simulink model "main_SEPETC"  (R2021a)
settings: Solver=VariableStepAuto  StartTime=0.0  StopTime=10  RelTol=1e-3
InitFcn:
  | run('Parameter.m')
values from neighbouring files (symbols this model uses):
  cp = 1    [Parameter.m]
  cv = 5    [Parameter.m]
  cw = 5    [Parameter.m]
  fref = 60    [Parameter.m]
  Lc1 = 0.35e-3    (= 0.00035)    [Parameter.m]
  Lc2 = 0.35e-3    (= 0.00035)    [Parameter.m]
  Lc3 = 0.35e-3    (= 0.00035)    [Parameter.m]
  Lc4 = 0.35e-3    (= 0.00035)    [Parameter.m]
  Lt12 = 318e-6    (= 0.000318)    [Parameter.m]
  Lt23 = 1847e-6    (= 0.001847)    [Parameter.m]
  Lt34 = 318e-6    (= 0.000318)    [Parameter.m]
  Mp1 = 9.4e-5    (= 9.4e-05)    [Parameter.m]
  Mp2 = 9.4e-5    (= 9.4e-05)    [Parameter.m]
  Mp3 = 12.5e-5    (= 0.000125)    [Parameter.m]
  Mp4 = 12.5e-5    (= 0.000125)    [Parameter.m]
  Nq1 = 1.3e-3    (= 0.0013)    [Parameter.m]
  Nq2 = 1.3e-3    (= 0.0013)    [Parameter.m]
  Nq3 = 1.5e-3    (= 0.0015)    [Parameter.m]
  Nq4 = 1.5e-3    (= 0.0015)    [Parameter.m]
  Rc1 = 0.03    [Parameter.m]
  Rc2 = 0.03    [Parameter.m]
  Rc3 = 0.03    [Parameter.m]
  Rc4 = 0.03    [Parameter.m]
  Rt12 = 0.23    [Parameter.m]
  Rt23 = 0.35    [Parameter.m]
  Rt34 = 0.23    [Parameter.m]
  t2 = 1    [Parameter.m]    (also in wvp_SEPETC.m)
  t3 = 10    [Parameter.m]
  t4 = 20    [Parameter.m]    (also in wvp_SEPETC.m = 21)
  t5 = 35    [Parameter.m]    (also in wvp_SEPETC.m = 33)
  t6 = 40    [Parameter.m]    (also in wvp_SEPETC.m = 35)
  Uo = 220*sqrt(2)    [Parameter.m]
  vref = 380    [Parameter.m]
  wc = 31.4    [Parameter.m]
  wref = 2*pi*fref    (= 376.991118431)    [Parameter.m]
undefined symbols (not defined in the file or in its folder): gcbh, sps_rtmsupport
libraries: spsControlledVoltageSourceLib x12, spsAlphaBetaZerotodq0Lib x12, eeGeneralControl x8, spsThreePhaseSeriesRLCBranchLib x7, spsGroundLib x4, spsThreePhaseVIMeasurementLib x4, spsThreePhaseBreakerLib x4, spsPLL3phLib x4, spsThreePhaseSeriesRLCLoadLib x3, spspowerguiLib x1
(part 2 of 3)

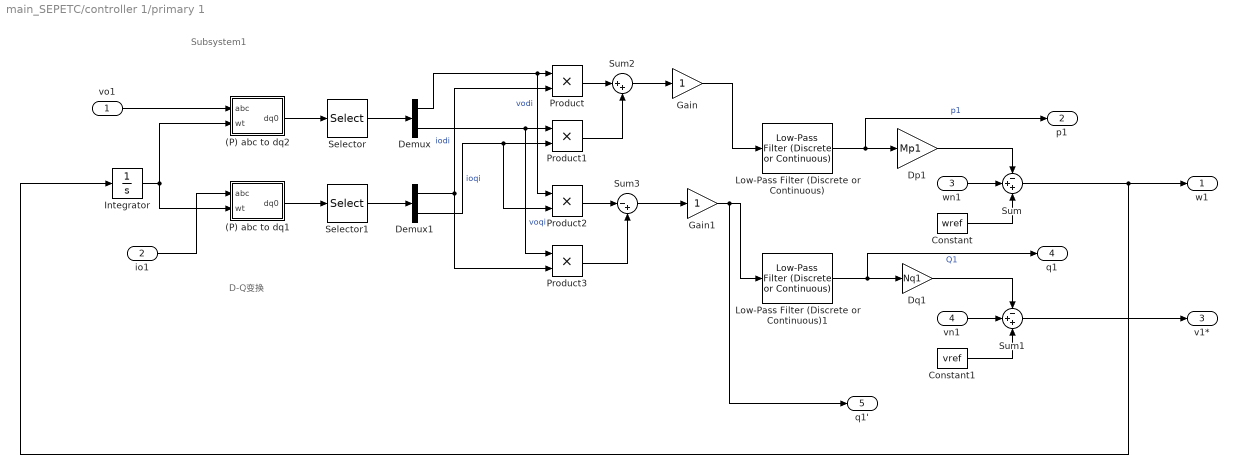
== system main_SEPETC/controller 1/primary 1 ==
  note: Subsystem1
  note: D-Q变换
  vo1 : Inport
  io1 : Inport  Port=2
  wn1 : Inport  Port=3
  vn1 : Inport  Port=4
  (P) abc to dq1 : Subsystem  AncestorBlock=powerlib_meascontrol/Transformations/abc to dq0  DialogController=POWERSYS.PowerSysDialog  LoadFcn=sps_rtmsupport('LoadFcn', gcbh);  StartFcn=sps_rtmsupport('StartFcn', gcbh);  StopFcn=sps_rtmsupport('StopFcn', gcbh);  mask(abc to dq0 Transformation){Alignment=90 degrees behind phase A axis}
      mask prompts: Alignment "Rotating frame alignment at wt=0:"
      mask help:
      | Perform a Park transformation from a three-phase (abc) signal to a dq0 rotating reference frame. Angular position of the rotating frame is given by input wt (rad).
      |
      | When the rotating frame alignment at wt=0 is 90 degrees behind phase A axis, a positive-sequence signal with Mag=1 & Phase=0 degrees yields the following dq values: d=1, q=0.
      mask init:
      | str=cat(2,gcb,'/Alpha-Beta-Zero to dq0');
      | if Alignment==1
      |     set_param(str,'Alignment','Aligned with phase A axis');
      | else
      |     set_param(str,'Alignment','90 degrees behind phase A axis');
      | end
      settings: CopyFcn=sps_rtmsupport('CopyFcn', gcbh);  DeleteFcn=sps_rtmsupport('DeleteFcn', gcbh);  UndoDeleteFcn=sps_rtmsupport('UndoDeleteFcn', gcbh);  ModelCloseFcn=sps_rtmsupport('ModelCloseFcn', gcbh);  PreSaveFcn=sps_rtmsupport('PreSaveFcn', gcbh);  PostSaveFcn=sps_rtmsupport('PostSaveFcn', gcbh);  NameChangeFcn=sps_rtmsupport('NameChangeFcn', gcbh);  PreCopyFcn=sps_rtmsupport('PreCopyFcn', gcbh);  OpenFcn=sps_rtmsupport('OpenFcn', gcbh, [1]);  CloseFcn=sps_rtmsupport('CloseFcn', gcbh);  PreDeleteFcn=sps_rtmsupport('PreDeleteFcn', gcbh);
      mask Help: helpview(psbhelp);
      mask TypeOptions Alignment: Aligned with phase A axis | 90 degrees behind phase A axis
      mask Display:
      | plot([0 1], [0,1])
      | port_label('input', 1, 'abc')
      | port_label('input', 2, 'wt')
      | port_label('output', 1, 'dq0')
  (P) abc to dq2 : Subsystem  AncestorBlock=powerlib_meascontrol/Transformations/abc to dq0  DialogController=POWERSYS.PowerSysDialog  LoadFcn=sps_rtmsupport('LoadFcn', gcbh);  StartFcn=sps_rtmsupport('StartFcn', gcbh);  StopFcn=sps_rtmsupport('StopFcn', gcbh);  mask(abc to dq0 Transformation){Alignment=90 degrees behind phase A axis}
      mask prompts: Alignment "Rotating frame alignment at wt=0:"
      mask help:
      | Perform a Park transformation from a three-phase (abc) signal to a dq0 rotating reference frame. Angular position of the rotating frame is given by input wt (rad).
      |
      | When the rotating frame alignment at wt=0 is 90 degrees behind phase A axis, a positive-sequence signal with Mag=1 & Phase=0 degrees yields the following dq values: d=1, q=0.
      mask init:
      | str=cat(2,gcb,'/Alpha-Beta-Zero to dq0');
      | if Alignment==1
      |     set_param(str,'Alignment','Aligned with phase A axis');
      | else
      |     set_param(str,'Alignment','90 degrees behind phase A axis');
      | end
      settings: CopyFcn=sps_rtmsupport('CopyFcn', gcbh);  DeleteFcn=sps_rtmsupport('DeleteFcn', gcbh);  UndoDeleteFcn=sps_rtmsupport('UndoDeleteFcn', gcbh);  ModelCloseFcn=sps_rtmsupport('ModelCloseFcn', gcbh);  PreSaveFcn=sps_rtmsupport('PreSaveFcn', gcbh);  PostSaveFcn=sps_rtmsupport('PostSaveFcn', gcbh);  NameChangeFcn=sps_rtmsupport('NameChangeFcn', gcbh);  PreCopyFcn=sps_rtmsupport('PreCopyFcn', gcbh);  OpenFcn=sps_rtmsupport('OpenFcn', gcbh, [1]);  CloseFcn=sps_rtmsupport('CloseFcn', gcbh);  PreDeleteFcn=sps_rtmsupport('PreDeleteFcn', gcbh);
      mask Help: helpview(psbhelp);
      mask TypeOptions Alignment: Aligned with phase A axis | 90 degrees behind phase A axis
      mask Display:
      | plot([0 1], [0,1])
      | port_label('input', 1, 'abc')
      | port_label('input', 2, 'wt')
      | port_label('output', 1, 'dq0')
  Constant : Constant  Value=wref
  Constant1 : Constant  Value=vref
  Demux : Demux  Outputs=2
  Demux1 : Demux  Outputs=2
  Dp1 : Gain  Gain=Mp1
  Dq1 : Gain  Gain=Nq1
  Gain : Gain
  Gain1 : Gain
  Integrator : Integrator
  Low-Pass Filter (Discrete or Continuous) : eeGeneralControl/Low-Pass Filter (Discrete or Continuous)  K=1  T=1/wc  B=inf  A=-inf  init_option=Inherited from block input  x0=0  Ts=-1
  Low-Pass Filter (Discrete or Continuous)1 : eeGeneralControl/Low-Pass Filter (Discrete or Continuous)  K=1  T=1/wc  B=inf  A=-inf  init_option=Inherited from block input  x0=0  Ts=-1
  Product{,1..3} (4 alike) : Product
  Selector : Selector  InputPortWidth=3  IndexOptions=Index vector (dialog)  Indices=[1 2]  OutputSizes=1
  Selector1 : Selector  InputPortWidth=3  IndexOptions=Index vector (dialog)  Indices=[1 2]  OutputSizes=1
  Sum : Sum  Inputs=-++
  Sum1 : Sum  Inputs=-++
  Sum2 : Sum  Inputs=|++
  Sum3 : Sum  Inputs=|-+
  w1 : Outport
  p1 : Outport  Port=2
  v1* : Outport  Port=3
  q1 : Outport  Port=4
  q1' : Outport  Port=5
  wires:
  Low-Pass Filter (Discrete or Continuous)/1 -> Dp1/1, p1/1  "p1"
  Dp1/1 -> Sum/1
  wn1/1 -> Sum/2
  Sum/1 -> Integrator/1, w1/1
  Dq1/1 -> Sum1/1
  Low-Pass Filter (Discrete or Continuous)1/1 -> Dq1/1, q1/1  "Q1"
  Sum1/1 -> v1*/1
  vn1/1 -> Sum1/2
  Constant1/1 -> Sum1/3
  Constant/1 -> Sum/3
  Gain1/1 -> q1'/1, Low-Pass Filter (Discrete or Continuous)1/1
  Gain/1 -> Low-Pass Filter (Discrete or Continuous)/1
  Sum3/1 -> Gain1/1
  Sum2/1 -> Gain/1
  vo1/1 -> (P) abc to dq2/1(abc)
  io1/1 -> (P) abc to dq1/1(abc)
  Product/1 -> Sum2/1
  Product1/1 -> Sum2/2
  Demux1/2 -> Product1/2, Product2/2  "ioqi"
  Product2/1 -> Sum3/1
  Product3/1 -> Sum3/2
  (P) abc to dq1/1(dq0) -> Selector1/1
  Demux1/1 -> Product3/2, Product/2  "iodi"
  (P) abc to dq2/1(dq0) -> Selector/1
  Demux/1 -> Product2/1, Product/1  "vodi"
  Integrator/1 -> (P) abc to dq1/2(wt), (P) abc to dq2/2(wt)
  Selector1/1 -> Demux1/1
  Demux/2 -> Product1/1, Product3/1  "voqi"
  Selector/1 -> Demux/1

== system main_SEPETC/controller 1/v_secondary 1 ==
  q1' : Inport
  Constant : Constant  Value=wc
  Gain1 : Gain  Gain=wc
  Gain11 : Gain  Gain=Nq1
  Gain5 : Gain  Gain=cv
  Integrator : Integrator  ExternalReset=rising
  Product : Product
  Step : Step  Time=t2  SampleTime=0
  Sum : Sum  Inputs=|+-
  Sum5 : Sum  Inputs=|++
  vn1 : Outport
  wires:
  [zv1] -> Gain5/1
  q1'/1 -> Product/1
  Constant/1 -> Product/2
  Product/1 -> Sum/1
  Gain1/1 -> Sum/2
  [q1] -> Gain1/1
  Sum/1 -> Gain11/1
  Gain5/1 -> Sum5/1
  Gain11/1 -> Sum5/2
  Sum5/1 -> Integrator/1
  Step/1 -> Integrator/2
  Integrator/1 -> vn1/1

== system main_SEPETC/controller 1/w_secondary 1 ==
  Gain : Gain  Gain=cw
  Gain15 : Gain  Gain=cp
  Integrator : Integrator  ExternalReset=rising
  Step : Step  Time=t2  SampleTime=0
  Sum6 : Sum  Inputs=++|
  wn1 : Outport
  wires:
  Sum6/1 -> Integrator/1
  Gain15/1 -> Sum6/2
  Integrator/1 -> wn1/1
  [zw1] -> Gain/1
  Gain/1 -> Sum6/1
  [zp1] -> Gain15/1
  Step/1 -> Integrator/2

== system main_SEPETC/controller 2/(P) abc to dq2 ==
  abc : Inport  PortDimensions=3
  wt : Inport  Port=2  PortDimensions=1
  Alpha-Beta-Zero to dq0 : spsAlphaBetaZerotodq0Lib/Alpha-Beta-Zero to dq0  Alignment=90 degrees behind phase A axis
      settings: SourceProductBaseCode=PS
  abc to Alpha-Beta-Zero : Subsystem  AncestorBlock=powerlib_meascontrol/Transformations/abc to Alpha-Beta-Zero  DialogController=POWERSYS.PowerSysDialog  LoadFcn=sps_rtmsupport('LoadFcn', gcbh);  StartFcn=sps_rtmsupport('StartFcn', gcbh);  StopFcn=sps_rtmsupport('StopFcn', gcbh);  mask(abc to Alpha-Beta-Zero Transformation){}
      mask help: Perform a Clarke transformation from a three-phase (abc) signal to a alpha-beta-zero stationary reference frame.
      settings: CopyFcn=sps_rtmsupport('CopyFcn', gcbh);  DeleteFcn=sps_rtmsupport('DeleteFcn', gcbh);  UndoDeleteFcn=sps_rtmsupport('UndoDeleteFcn', gcbh);  ModelCloseFcn=sps_rtmsupport('ModelCloseFcn', gcbh);  PreSaveFcn=sps_rtmsupport('PreSaveFcn', gcbh);  PostSaveFcn=sps_rtmsupport('PostSaveFcn', gcbh);  NameChangeFcn=sps_rtmsupport('NameChangeFcn', gcbh);  PreCopyFcn=sps_rtmsupport('PreCopyFcn', gcbh);  OpenFcn=sps_rtmsupport('OpenFcn', gcbh, []);  CloseFcn=sps_rtmsupport('CloseFcn', gcbh);  PreDeleteFcn=sps_rtmsupport('PreDeleteFcn', gcbh);
      mask Help: helpview(psbhelp);
      mask Display:
      | plot([0 1], [0,1])
      | text(0.15,0.7,'abc')
      | text(0.55, 0.3,'\alpha\beta0','texmode','on')
  dq0 : Outport  VectorParamsAs1DForOutWhenUnconnected=off
  wires:
  wt/1 -> Alpha-Beta-Zero to dq0/2
  abc/1 -> abc to Alpha-Beta-Zero/1(abc)
  Alpha-Beta-Zero to dq0/1 -> dq0/1
  abc to Alpha-Beta-Zero/1(al_be_0) -> Alpha-Beta-Zero to dq0/1

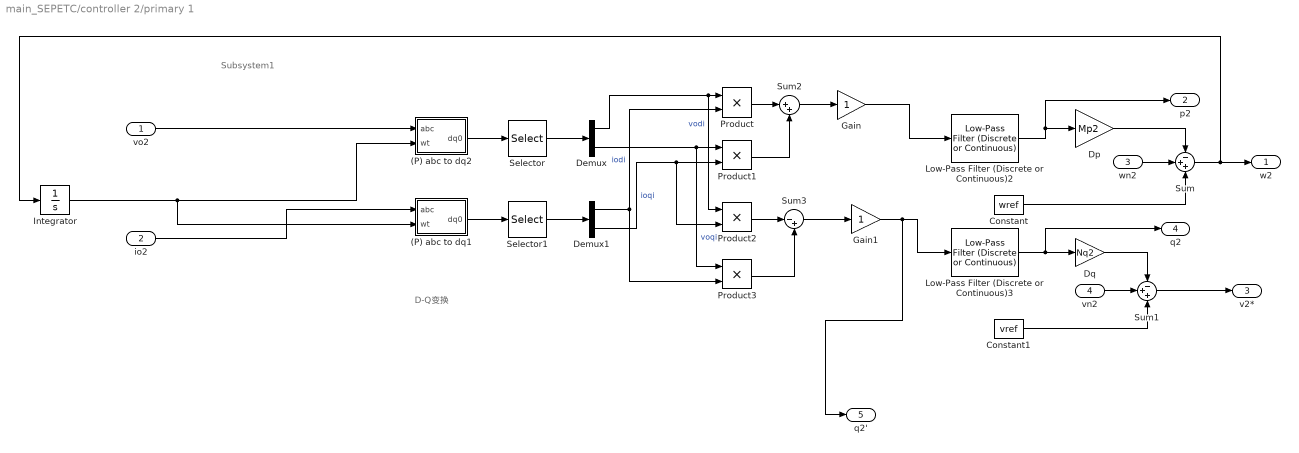
== system main_SEPETC/controller 2/primary 1 ==
  note: Subsystem1
  note: D-Q变换
  vo2 : Inport
  io2 : Inport  Port=2
  wn2 : Inport  Port=3
  vn2 : Inport  Port=4
  (P) abc to dq1 : Subsystem  AncestorBlock=powerlib_meascontrol/Transformations/abc to dq0  DialogController=POWERSYS.PowerSysDialog  LoadFcn=sps_rtmsupport('LoadFcn', gcbh);  StartFcn=sps_rtmsupport('StartFcn', gcbh);  StopFcn=sps_rtmsupport('StopFcn', gcbh);  mask(abc to dq0 Transformation){Alignment=90 degrees behind phase A axis}
      mask prompts: Alignment "Rotating frame alignment at wt=0:"
      mask help:
      | Perform a Park transformation from a three-phase (abc) signal to a dq0 rotating reference frame. Angular position of the rotating frame is given by input wt (rad).
      |
      | When the rotating frame alignment at wt=0 is 90 degrees behind phase A axis, a positive-sequence signal with Mag=1 & Phase=0 degrees yields the following dq values: d=1, q=0.
      mask init:
      | str=cat(2,gcb,'/Alpha-Beta-Zero to dq0');
      | if Alignment==1
      |     set_param(str,'Alignment','Aligned with phase A axis');
      | else
      |     set_param(str,'Alignment','90 degrees behind phase A axis');
      | end
      settings: CopyFcn=sps_rtmsupport('CopyFcn', gcbh);  DeleteFcn=sps_rtmsupport('DeleteFcn', gcbh);  UndoDeleteFcn=sps_rtmsupport('UndoDeleteFcn', gcbh);  ModelCloseFcn=sps_rtmsupport('ModelCloseFcn', gcbh);  PreSaveFcn=sps_rtmsupport('PreSaveFcn', gcbh);  PostSaveFcn=sps_rtmsupport('PostSaveFcn', gcbh);  NameChangeFcn=sps_rtmsupport('NameChangeFcn', gcbh);  PreCopyFcn=sps_rtmsupport('PreCopyFcn', gcbh);  OpenFcn=sps_rtmsupport('OpenFcn', gcbh, [1]);  CloseFcn=sps_rtmsupport('CloseFcn', gcbh);  PreDeleteFcn=sps_rtmsupport('PreDeleteFcn', gcbh);
      mask Help: helpview(psbhelp);
      mask TypeOptions Alignment: Aligned with phase A axis | 90 degrees behind phase A axis
      mask Display:
      | plot([0 1], [0,1])
      | port_label('input', 1, 'abc')
      | port_label('input', 2, 'wt')
      | port_label('output', 1, 'dq0')
  (P) abc to dq2 : Subsystem  AncestorBlock=powerlib_meascontrol/Transformations/abc to dq0  DialogController=POWERSYS.PowerSysDialog  LoadFcn=sps_rtmsupport('LoadFcn', gcbh);  StartFcn=sps_rtmsupport('StartFcn', gcbh);  StopFcn=sps_rtmsupport('StopFcn', gcbh);  mask(abc to dq0 Transformation){Alignment=90 degrees behind phase A axis}
      mask prompts: Alignment "Rotating frame alignment at wt=0:"
      mask help:
      | Perform a Park transformation from a three-phase (abc) signal to a dq0 rotating reference frame. Angular position of the rotating frame is given by input wt (rad).
      |
      | When the rotating frame alignment at wt=0 is 90 degrees behind phase A axis, a positive-sequence signal with Mag=1 & Phase=0 degrees yields the following dq values: d=1, q=0.
      mask init:
      | str=cat(2,gcb,'/Alpha-Beta-Zero to dq0');
      | if Alignment==1
      |     set_param(str,'Alignment','Aligned with phase A axis');
      | else
      |     set_param(str,'Alignment','90 degrees behind phase A axis');
      | end
      settings: CopyFcn=sps_rtmsupport('CopyFcn', gcbh);  DeleteFcn=sps_rtmsupport('DeleteFcn', gcbh);  UndoDeleteFcn=sps_rtmsupport('UndoDeleteFcn', gcbh);  ModelCloseFcn=sps_rtmsupport('ModelCloseFcn', gcbh);  PreSaveFcn=sps_rtmsupport('PreSaveFcn', gcbh);  PostSaveFcn=sps_rtmsupport('PostSaveFcn', gcbh);  NameChangeFcn=sps_rtmsupport('NameChangeFcn', gcbh);  PreCopyFcn=sps_rtmsupport('PreCopyFcn', gcbh);  OpenFcn=sps_rtmsupport('OpenFcn', gcbh, [1]);  CloseFcn=sps_rtmsupport('CloseFcn', gcbh);  PreDeleteFcn=sps_rtmsupport('PreDeleteFcn', gcbh);
      mask Help: helpview(psbhelp);
      mask TypeOptions Alignment: Aligned with phase A axis | 90 degrees behind phase A axis
      mask Display:
      | plot([0 1], [0,1])
      | port_label('input', 1, 'abc')
      | port_label('input', 2, 'wt')
      | port_label('output', 1, 'dq0')
  Constant : Constant  Value=wref
  Constant1 : Constant  Value=vref
  Demux : Demux  Outputs=2
  Demux1 : Demux  Outputs=2
  Dp : Gain  Gain=Mp2
  Dq : Gain  Gain=Nq2
  Gain : Gain
  Gain1 : Gain
  Integrator : Integrator
  Low-Pass Filter (Discrete or Continuous)2 : eeGeneralControl/Low-Pass Filter (Discrete or Continuous)  K=1  T=1/wc  B=inf  A=-inf  init_option=Inherited from block input  x0=0  Ts=-1
  Low-Pass Filter (Discrete or Continuous)3 : eeGeneralControl/Low-Pass Filter (Discrete or Continuous)  K=1  T=1/wc  B=inf  A=-inf  init_option=Inherited from block input  x0=0  Ts=-1
  Product{,1..3} (4 alike) : Product
  Selector : Selector  InputPortWidth=3  IndexOptions=Index vector (dialog)  Indices=[1 2]  OutputSizes=1
  Selector1 : Selector  InputPortWidth=3  IndexOptions=Index vector (dialog)  Indices=[1 2]  OutputSizes=1
  Sum : Sum  Inputs=-++
  Sum1 : Sum  Inputs=-++
  Sum2 : Sum  Inputs=|++
  Sum3 : Sum  Inputs=|-+
  w2 : Outport
  p2 : Outport  Port=2
  v2* : Outport  Port=3
  q2 : Outport  Port=4
  q2' : Outport  Port=5
  wires:
  vn2/1 -> Sum1/2
  Constant/1 -> Sum/3
  Sum1/1 -> v2*/1
  Constant1/1 -> Sum1/3
  Low-Pass Filter (Discrete or Continuous)3/1 -> Dq/1, q2/1
  Sum/1 -> w2/1, Integrator/1
  Dq/1 -> Sum1/1
  wn2/1 -> Sum/2
  Dp/1 -> Sum/1
  Low-Pass Filter (Discrete or Continuous)2/1 -> Dp/1, p2/1
  Gain1/1 -> q2'/1, Low-Pass Filter (Discrete or Continuous)3/1
  Gain/1 -> Low-Pass Filter (Discrete or Continuous)2/1
  Sum3/1 -> Gain1/1
  Sum2/1 -> Gain/1
  vo2/1 -> (P) abc to dq2/1(abc)
  io2/1 -> (P) abc to dq1/1(abc)
  Product/1 -> Sum2/1
  Product1/1 -> Sum2/2
  Demux1/2 -> Product1/2, Product2/2  "ioqi"
  Product2/1 -> Sum3/1
  Product3/1 -> Sum3/2
  (P) abc to dq1/1(dq0) -> Selector1/1
  Demux1/1 -> Product3/2, Product/2  "iodi"
  (P) abc to dq2/1(dq0) -> Selector/1
  Demux/1 -> Product2/1, Product/1  "vodi"
  Integrator/1 -> (P) abc to dq1/2(wt), (P) abc to dq2/2(wt)
  Selector1/1 -> Demux1/1
  Demux/2 -> Product1/1, Product3/1  "voqi"
  Selector/1 -> Demux/1

== system main_SEPETC/controller 2/v_secondary 2 ==
  q2' : Inport
  Constant : Constant  Value=wc
  Gain1 : Gain  Gain=wc
  Gain11 : Gain  Gain=Nq2
  Gain5 : Gain  Gain=cv
  Integrator2 : Integrator  ExternalReset=rising
  Product : Product
  Step : Step  Time=t2  SampleTime=0
  Sum : Sum  Inputs=|+-
  Sum6 : Sum  Inputs=++|
  vn2 : Outport
  wires:
  [zv2] -> Gain5/1
  Sum/1 -> Gain11/1
  [q2] -> Gain1/1
  Gain11/1 -> Sum6/2
  Product/1 -> Sum/1
  q2'/1 -> Product/1
  Gain1/1 -> Sum/2
  Constant/1 -> Product/2
  Gain5/1 -> Sum6/1
  Sum6/1 -> Integrator2/1
  Step/1 -> Integrator2/2
  Integrator2/1 -> vn2/1

== system main_SEPETC/controller 2/w_secondary 2 ==
  Gain : Gain  Gain=cw
  Gain15 : Gain  Gain=cp
  Integrator : Integrator  ExternalReset=rising
  Step : Step  Time=t2  SampleTime=0
  Sum1 : Sum  Inputs=++|
  wn2 : Outport
  wires:
  [zp2] -> Gain15/1
  Integrator/1 -> wn2/1
  Gain15/1 -> Sum1/2
  [zw2] -> Gain/1
  Gain/1 -> Sum1/1
  Step/1 -> Integrator/2
  Sum1/1 -> Integrator/1

== system main_SEPETC/controller 3/(P) abc to dq2 ==
  abc : Inport  PortDimensions=3
  wt : Inport  Port=2  PortDimensions=1
  Alpha-Beta-Zero to dq0 : spsAlphaBetaZerotodq0Lib/Alpha-Beta-Zero to dq0  Alignment=90 degrees behind phase A axis
      settings: SourceProductBaseCode=PS
  abc to Alpha-Beta-Zero : Subsystem  AncestorBlock=powerlib_meascontrol/Transformations/abc to Alpha-Beta-Zero  DialogController=POWERSYS.PowerSysDialog  LoadFcn=sps_rtmsupport('LoadFcn', gcbh);  StartFcn=sps_rtmsupport('StartFcn', gcbh);  StopFcn=sps_rtmsupport('StopFcn', gcbh);  mask(abc to Alpha-Beta-Zero Transformation){}
      mask help: Perform a Clarke transformation from a three-phase (abc) signal to a alpha-beta-zero stationary reference frame.
      settings: CopyFcn=sps_rtmsupport('CopyFcn', gcbh);  DeleteFcn=sps_rtmsupport('DeleteFcn', gcbh);  UndoDeleteFcn=sps_rtmsupport('UndoDeleteFcn', gcbh);  ModelCloseFcn=sps_rtmsupport('ModelCloseFcn', gcbh);  PreSaveFcn=sps_rtmsupport('PreSaveFcn', gcbh);  PostSaveFcn=sps_rtmsupport('PostSaveFcn', gcbh);  NameChangeFcn=sps_rtmsupport('NameChangeFcn', gcbh);  PreCopyFcn=sps_rtmsupport('PreCopyFcn', gcbh);  OpenFcn=sps_rtmsupport('OpenFcn', gcbh, []);  CloseFcn=sps_rtmsupport('CloseFcn', gcbh);  PreDeleteFcn=sps_rtmsupport('PreDeleteFcn', gcbh);
      mask Help: helpview(psbhelp);
      mask Display:
      | plot([0 1], [0,1])
      | text(0.15,0.7,'abc')
      | text(0.55, 0.3,'\alpha\beta0','texmode','on')
  dq0 : Outport  VectorParamsAs1DForOutWhenUnconnected=off
  wires:
  wt/1 -> Alpha-Beta-Zero to dq0/2
  abc/1 -> abc to Alpha-Beta-Zero/1(abc)
  Alpha-Beta-Zero to dq0/1 -> dq0/1
  abc to Alpha-Beta-Zero/1(al_be_0) -> Alpha-Beta-Zero to dq0/1

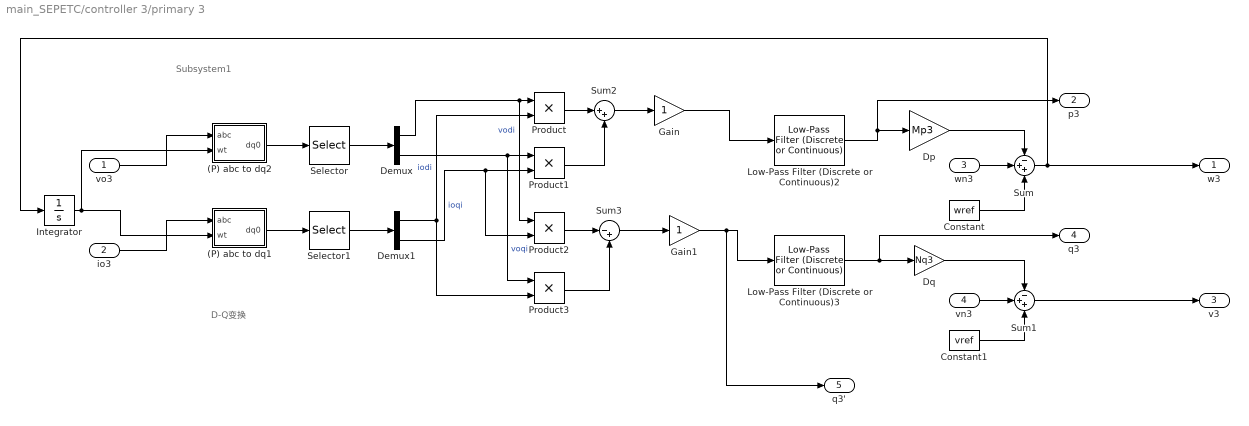
== system main_SEPETC/controller 3/primary 3 ==
  note: Subsystem1
  note: D-Q变换
  vo3 : Inport
  io3 : Inport  Port=2
  wn3 : Inport  Port=3
  vn3 : Inport  Port=4
  (P) abc to dq1 : Subsystem  AncestorBlock=powerlib_meascontrol/Transformations/abc to dq0  DialogController=POWERSYS.PowerSysDialog  LoadFcn=sps_rtmsupport('LoadFcn', gcbh);  StartFcn=sps_rtmsupport('StartFcn', gcbh);  StopFcn=sps_rtmsupport('StopFcn', gcbh);  mask(abc to dq0 Transformation){Alignment=90 degrees behind phase A axis}
      mask prompts: Alignment "Rotating frame alignment at wt=0:"
      mask help:
      | Perform a Park transformation from a three-phase (abc) signal to a dq0 rotating reference frame. Angular position of the rotating frame is given by input wt (rad).
      |
      | When the rotating frame alignment at wt=0 is 90 degrees behind phase A axis, a positive-sequence signal with Mag=1 & Phase=0 degrees yields the following dq values: d=1, q=0.
      mask init:
      | str=cat(2,gcb,'/Alpha-Beta-Zero to dq0');
      | if Alignment==1
      |     set_param(str,'Alignment','Aligned with phase A axis');
      | else
      |     set_param(str,'Alignment','90 degrees behind phase A axis');
      | end
      settings: CopyFcn=sps_rtmsupport('CopyFcn', gcbh);  DeleteFcn=sps_rtmsupport('DeleteFcn', gcbh);  UndoDeleteFcn=sps_rtmsupport('UndoDeleteFcn', gcbh);  ModelCloseFcn=sps_rtmsupport('ModelCloseFcn', gcbh);  PreSaveFcn=sps_rtmsupport('PreSaveFcn', gcbh);  PostSaveFcn=sps_rtmsupport('PostSaveFcn', gcbh);  NameChangeFcn=sps_rtmsupport('NameChangeFcn', gcbh);  PreCopyFcn=sps_rtmsupport('PreCopyFcn', gcbh);  OpenFcn=sps_rtmsupport('OpenFcn', gcbh, [1]);  CloseFcn=sps_rtmsupport('CloseFcn', gcbh);  PreDeleteFcn=sps_rtmsupport('PreDeleteFcn', gcbh);
      mask Help: helpview(psbhelp);
      mask TypeOptions Alignment: Aligned with phase A axis | 90 degrees behind phase A axis
      mask Display:
      | plot([0 1], [0,1])
      | port_label('input', 1, 'abc')
      | port_label('input', 2, 'wt')
      | port_label('output', 1, 'dq0')
  (P) abc to dq2 : Subsystem  AncestorBlock=powerlib_meascontrol/Transformations/abc to dq0  DialogController=POWERSYS.PowerSysDialog  LoadFcn=sps_rtmsupport('LoadFcn', gcbh);  StartFcn=sps_rtmsupport('StartFcn', gcbh);  StopFcn=sps_rtmsupport('StopFcn', gcbh);  mask(abc to dq0 Transformation){Alignment=90 degrees behind phase A axis}
      mask prompts: Alignment "Rotating frame alignment at wt=0:"
      mask help:
      | Perform a Park transformation from a three-phase (abc) signal to a dq0 rotating reference frame. Angular position of the rotating frame is given by input wt (rad).
      |
      | When the rotating frame alignment at wt=0 is 90 degrees behind phase A axis, a positive-sequence signal with Mag=1 & Phase=0 degrees yields the following dq values: d=1, q=0.
      mask init:
      | str=cat(2,gcb,'/Alpha-Beta-Zero to dq0');
      | if Alignment==1
      |     set_param(str,'Alignment','Aligned with phase A axis');
      | else
      |     set_param(str,'Alignment','90 degrees behind phase A axis');
      | end
      settings: CopyFcn=sps_rtmsupport('CopyFcn', gcbh);  DeleteFcn=sps_rtmsupport('DeleteFcn', gcbh);  UndoDeleteFcn=sps_rtmsupport('UndoDeleteFcn', gcbh);  ModelCloseFcn=sps_rtmsupport('ModelCloseFcn', gcbh);  PreSaveFcn=sps_rtmsupport('PreSaveFcn', gcbh);  PostSaveFcn=sps_rtmsupport('PostSaveFcn', gcbh);  NameChangeFcn=sps_rtmsupport('NameChangeFcn', gcbh);  PreCopyFcn=sps_rtmsupport('PreCopyFcn', gcbh);  OpenFcn=sps_rtmsupport('OpenFcn', gcbh, [1]);  CloseFcn=sps_rtmsupport('CloseFcn', gcbh);  PreDeleteFcn=sps_rtmsupport('PreDeleteFcn', gcbh);
      mask Help: helpview(psbhelp);
      mask TypeOptions Alignment: Aligned with phase A axis | 90 degrees behind phase A axis
      mask Display:
      | plot([0 1], [0,1])
      | port_label('input', 1, 'abc')
      | port_label('input', 2, 'wt')
      | port_label('output', 1, 'dq0')
  Constant : Constant  Value=wref
  Constant1 : Constant  Value=vref
  Demux : Demux  Outputs=2
  Demux1 : Demux  Outputs=2
  Dp : Gain  Gain=Mp3
  Dq : Gain  Gain=Nq3
  Gain : Gain
  Gain1 : Gain
  Integrator : Integrator
  Low-Pass Filter (Discrete or Continuous)2 : eeGeneralControl/Low-Pass Filter (Discrete or Continuous)  K=1  T=1/wc  B=inf  A=-inf  init_option=Inherited from block input  x0=0  Ts=-1
  Low-Pass Filter (Discrete or Continuous)3 : eeGeneralControl/Low-Pass Filter (Discrete or Continuous)  K=1  T=1/wc  B=inf  A=-inf  init_option=Inherited from block input  x0=0  Ts=-1
  Product{,1..3} (4 alike) : Product
  Selector : Selector  InputPortWidth=3  IndexOptions=Index vector (dialog)  Indices=[1 2]  OutputSizes=1
  Selector1 : Selector  InputPortWidth=3  IndexOptions=Index vector (dialog)  Indices=[1 2]  OutputSizes=1
  Sum : Sum  Inputs=-++
  Sum1 : Sum  Inputs=-++
  Sum2 : Sum  Inputs=|++
  Sum3 : Sum  Inputs=|-+
  w3 : Outport
  p3 : Outport  Port=2
  v3 : Outport  Port=3
  q3 : Outport  Port=4
  q3' : Outport  Port=5
  wires:
  vn3/1 -> Sum1/2
  Constant/1 -> Sum/3
  Sum1/1 -> v3/1
  Constant1/1 -> Sum1/3
  Low-Pass Filter (Discrete or Continuous)3/1 -> Dq/1, q3/1
  Sum/1 -> w3/1, Integrator/1
  Dq/1 -> Sum1/1
  wn3/1 -> Sum/2
  Dp/1 -> Sum/1
  Low-Pass Filter (Discrete or Continuous)2/1 -> Dp/1, p3/1
  Gain1/1 -> Low-Pass Filter (Discrete or Continuous)3/1, q3'/1
  Gain/1 -> Low-Pass Filter (Discrete or Continuous)2/1
  Sum3/1 -> Gain1/1
  Sum2/1 -> Gain/1
  vo3/1 -> (P) abc to dq2/1(abc)
  io3/1 -> (P) abc to dq1/1(abc)
  Product/1 -> Sum2/1
  Product1/1 -> Sum2/2
  Demux1/2 -> Product1/2, Product2/2  "ioqi"
  Product2/1 -> Sum3/1
  Product3/1 -> Sum3/2
  (P) abc to dq1/1(dq0) -> Selector1/1
  Demux1/1 -> Product3/2, Product/2  "iodi"
  (P) abc to dq2/1(dq0) -> Selector/1
  Demux/1 -> Product2/1, Product/1  "vodi"
  Integrator/1 -> (P) abc to dq1/2(wt), (P) abc to dq2/2(wt)
  Selector1/1 -> Demux1/1
  Demux/2 -> Product1/1, Product3/1  "voqi"
  Selector/1 -> Demux/1

== system main_SEPETC/controller 3/v_secondary 3 ==
  q3' : Inport
  Constant : Constant  Value=wc
  Gain1 : Gain  Gain=wc
  Gain11 : Gain  Gain=Nq3
  Gain5 : Gain  Gain=cv
  Integrator2 : Integrator  ExternalReset=rising
  Product : Product
  Subsystem2 : Subsystem
  Sum : Sum  Inputs=|+-
  Sum1 : Sum  Inputs=++|
  vn3 : Outport
  wires:
  [zv3] -> Gain5/1
  Gain5/1 -> Sum1/1
  Integrator2/1 -> vn3/1
  Gain11/1 -> Sum1/2
  Gain1/1 -> Sum/2
  Constant/1 -> Product/2
  q3'/1 -> Product/1
  [q3] -> Gain1/1
  Product/1 -> Sum/1
  Sum/1 -> Gain11/1
  [t] -> Integrator2/2
  Sum1/1 -> Subsystem2/1(In1)
  Subsystem2/1(Out1) -> Integrator2/1

== system main_SEPETC/controller 3/w_secondary 3 ==
  Gain1 : Gain  Gain=cw
  Gain15 : Gain  Gain=cp
  Integrator : Integrator  ExternalReset=rising
  Subsystem2 : Subsystem
  Sum6 : Sum  Inputs=++|
  wn3 : Outport
  wires:
  Integrator/1 -> wn3/1
  Gain15/1 -> Sum6/2
  [zw3] -> Gain1/1
  Gain1/1 -> Sum6/1
  [zp3] -> Gain15/1
  [t] -> Integrator/2
  Sum6/1 -> Subsystem2/1(In1)
  Subsystem2/1(Out1) -> Integrator/1

== system main_SEPETC/controller 4/(P) abc to dq2 ==
  abc : Inport  PortDimensions=3
  wt : Inport  Port=2  PortDimensions=1
  Alpha-Beta-Zero to dq0 : spsAlphaBetaZerotodq0Lib/Alpha-Beta-Zero to dq0  Alignment=90 degrees behind phase A axis
      settings: SourceProductBaseCode=PS
  abc to Alpha-Beta-Zero : Subsystem  AncestorBlock=powerlib_meascontrol/Transformations/abc to Alpha-Beta-Zero  DialogController=POWERSYS.PowerSysDialog  LoadFcn=sps_rtmsupport('LoadFcn', gcbh);  StartFcn=sps_rtmsupport('StartFcn', gcbh);  StopFcn=sps_rtmsupport('StopFcn', gcbh);  mask(abc to Alpha-Beta-Zero Transformation){}
      mask help: Perform a Clarke transformation from a three-phase (abc) signal to a alpha-beta-zero stationary reference frame.
      settings: CopyFcn=sps_rtmsupport('CopyFcn', gcbh);  DeleteFcn=sps_rtmsupport('DeleteFcn', gcbh);  UndoDeleteFcn=sps_rtmsupport('UndoDeleteFcn', gcbh);  ModelCloseFcn=sps_rtmsupport('ModelCloseFcn', gcbh);  PreSaveFcn=sps_rtmsupport('PreSaveFcn', gcbh);  PostSaveFcn=sps_rtmsupport('PostSaveFcn', gcbh);  NameChangeFcn=sps_rtmsupport('NameChangeFcn', gcbh);  PreCopyFcn=sps_rtmsupport('PreCopyFcn', gcbh);  OpenFcn=sps_rtmsupport('OpenFcn', gcbh, []);  CloseFcn=sps_rtmsupport('CloseFcn', gcbh);  PreDeleteFcn=sps_rtmsupport('PreDeleteFcn', gcbh);
      mask Help: helpview(psbhelp);
      mask Display:
      | plot([0 1], [0,1])
      | text(0.15,0.7,'abc')
      | text(0.55, 0.3,'\alpha\beta0','texmode','on')
  dq0 : Outport  VectorParamsAs1DForOutWhenUnconnected=off
  wires:
  wt/1 -> Alpha-Beta-Zero to dq0/2
  abc/1 -> abc to Alpha-Beta-Zero/1(abc)
  Alpha-Beta-Zero to dq0/1 -> dq0/1
  abc to Alpha-Beta-Zero/1(al_be_0) -> Alpha-Beta-Zero to dq0/1

== system main_SEPETC/controller 4/primary 3 ==
  vo4 : Inport
  io4 : Inport  Port=2
  wn4 : Inport  Port=3
  vn4 : Inport  Port=4
  Constant : Constant  Value=wref
  Constant1 : Constant  Value=vref
  Dp : Gain  Gain=Mp4
  Dq : Gain  Gain=Nq4
  Integrator : Integrator
  Low-Pass Filter (Discrete or Continuous)2 : eeGeneralControl/Low-Pass Filter (Discrete or Continuous)  K=1  T=1/wc  B=inf  A=-inf  init_option=Inherited from block input  x0=0  Ts=-1
  Low-Pass Filter (Discrete or Continuous)3 : eeGeneralControl/Low-Pass Filter (Discrete or Continuous)  K=1  T=1/wc  B=inf  A=-inf  init_option=Inherited from block input  x0=0  Ts=-1
  Subsystem1 : Subsystem
  Sum : Sum  Inputs=-++
  Sum1 : Sum  Inputs=-++
  w4 : Outport
  p4 : Outport  Port=2
  v4 : Outport  Port=3
  q4 : Outport  Port=4
  q4' : Outport  Port=5
  wires:
  vn4/1 -> Sum1/2
  Constant/1 -> Sum/3
  Sum1/1 -> v4/1
  Constant1/1 -> Sum1/3
  Low-Pass Filter (Discrete or Continuous)3/1 -> Dq/1, q4/1
  Sum/1 -> w4/1, Integrator/1
  Dq/1 -> Sum1/1
  wn4/1 -> Sum/2
  Dp/1 -> Sum/1
  Low-Pass Filter (Discrete or Continuous)2/1 -> Dp/1, p4/1
  Subsystem1/2(q') -> Low-Pass Filter (Discrete or Continuous)3/1, q4'/1
  vo4/1 -> Subsystem1/1(Vo1)
  Integrator/1 -> Subsystem1/2(wt)
  io4/1 -> Subsystem1/3(io1)
  Subsystem1/1(p') -> Low-Pass Filter (Discrete or Continuous)2/1

== system main_SEPETC/controller 4/v_secondary 4 ==
  q4' : Inport
  Constant : Constant  Value=wc
  Gain1 : Gain  Gain=wc
  Gain11 : Gain  Gain=Nq4
  Gain5 : Gain  Gain=cv
  Integrator2 : Integrator  ExternalReset=rising
  Product : Product
  Step : Step  Time=t2  SampleTime=0
  Sum : Sum  Inputs=|+-
  Sum6 : Sum  Inputs=++|
  vn4 : Outport
  wires:
  [zv4] -> Gain5/1
  Integrator2/1 -> vn4/1
  Gain11/1 -> Sum6/2
  Sum6/1 -> Integrator2/1
  Gain1/1 -> Sum/2
  Constant/1 -> Product/2
  q4'/1 -> Product/1
  [q4] -> Gain1/1
  Product/1 -> Sum/1
  Sum/1 -> Gain11/1
  Step/1 -> Integrator2/2
  Gain5/1 -> Sum6/1

== system main_SEPETC/controller 4/w_secondary 4 ==
  Gain1 : Gain  Gain=cw
  Gain15 : Gain  Gain=cp
  Integrator : Integrator  ExternalReset=rising
  Step : Step  Time=t2  SampleTime=0
  Sum6 : Sum  Inputs=++|
  wn4 : Outport
  wires:
  Integrator/1 -> wn4/1
  Sum6/1 -> Integrator/1
  Gain15/1 -> Sum6/2
  [zw4] -> Gain1/1
  Gain1/1 -> Sum6/1
  [zp4] -> Gain15/1
  Step/1 -> Integrator/2

== system main_SEPETC/active power sharing SE-PETC /EState_1/x1_o1 ==
  Gain : Gain  Gain=cp
  Integrator : Integrator  ExternalReset=rising
  Sum : Sum  Inputs=|+-
  Sum2 : Sum  Inputs=|++
  Sum3 : Sum  Inputs=|++
  Sum4 : Sum  Inputs=|+-
  x1_o1 : Outport
  wires:
  Integrator/1 -> Sum3/1
  [x1_hat] -> Sum3/2
  [flag1] -> Integrator/2
  Sum2/1 -> Gain/1
  Gain/1 -> Integrator/1
  [x1_o2_hat] -> Sum/1
  [x1_o4_hat] -> Sum4/1
  Sum3/1 -> Sum/2, Sum4/2, x1_o1/1
  Sum/1 -> Sum2/2
  Sum4/1 -> Sum2/1

== system main_SEPETC/active power sharing SE-PETC /EState_1/x1_o2 ==
  note: 利用x2对邻居的观测值，估计x2的状态
  Gain : Gain  Gain=cp
  Integrator : Integrator  ExternalReset=rising
  Subsystem1 : Subsystem
  Sum : Sum  Inputs=|+-
  Sum2 : Sum  Inputs=|++
  Sum3 : Sum  Inputs=|++
  Sum4 : Sum  Inputs=|+-
  x1_o2 : Outport
  wires:
  Sum/1 -> Sum2/1
  Integrator/1 -> Sum3/1
  Sum3/1 -> Sum4/2, Sum/2, x1_o2/1
  [flag2] -> Integrator/2
  Sum2/1 -> Gain/1
  Gain/1 -> Integrator/1
  [x2_o3_hat] -> Sum4/1
  [x2_o1_hat] -> Sum/1
  [x2_hat] -> Sum3/2
  Sum4/1 -> Subsystem1/1(In1)
  Subsystem1/1(Out1) -> Sum2/2

== system main_SEPETC/active power sharing SE-PETC /EState_1/x1_o4 ==
  note: 利用x4对邻居的观测值，估计x4的状态
  Gain : Gain  Gain=cp
  Integrator : Integrator  ExternalReset=rising
  Subsystem4 : Subsystem
  Sum : Sum  Inputs=|+-
  Sum2 : Sum  Inputs=|++
  Sum3 : Sum  Inputs=|++
  Sum4 : Sum  Inputs=|+-
  x1_o4 : Outport
  wires:
  Sum/1 -> Sum2/1
  Integrator/1 -> Sum3/1
  Sum3/1 -> x1_o4/1, Sum4/2, Sum/2
  Gain/1 -> Integrator/1
  [x4_o3_hat] -> Sum4/1
  [x4_o1_hat] -> Sum/1
  Sum2/1 -> Gain/1
  [x4_hat] -> Sum3/2
  [flag4] -> Integrator/2
  Sum4/1 -> Subsystem4/1(In1)
  Subsystem4/1(Out1) -> Sum2/2

== system main_SEPETC/active power sharing SE-PETC /EState_2/x2_o1 ==
  note: 利用x1对邻居的观测值，估计x1的状态
  Gain1 : Gain  Gain=cp
  Integrator1 : Integrator  ExternalReset=rising
  Sum4 : Sum  Inputs=|+-
  Sum6 : Sum  Inputs=|++
  Sum7 : Sum  Inputs=|++
  Sum8 : Sum  Inputs=|+-
  x2_o1 : Outport
  wires:
  Sum7/1 -> Sum8/2, Sum4/2, x2_o1/1
  Sum8/1 -> Sum6/2
  [x1_o2_hat] -> Sum4/1
  [x1_o4_hat] -> Sum8/1
  Integrator1/1 -> Sum7/1
  Sum6/1 -> Gain1/1
  [flag1] -> Integrator1/2
  Gain1/1 -> Integrator1/1
  [x1_hat] -> Sum7/2
  Sum4/1 -> Sum6/1

== system main_SEPETC/active power sharing SE-PETC /EState_2/x2_o2 ==
  Gain : Gain  Gain=cp
  Integrator : Integrator  ExternalReset=rising
  Subsystem1 : Subsystem
  Sum : Sum  Inputs=|+-
  Sum2 : Sum  Inputs=|++
  Sum3 : Sum  Inputs=|++
  Sum4 : Sum  Inputs=|+-
  x2_o2 : Outport
  wires:
  Sum/1 -> Sum2/1
  Integrator/1 -> Sum3/1
  [x2_hat] -> Sum3/2
  Sum3/1 -> Sum4/2, Sum/2, x2_o2/1
  [flag2] -> Integrator/2
  Sum2/1 -> Gain/1
  Gain/1 -> Integrator/1
  [x2_o1_hat] -> Sum/1
  [x2_o3_hat] -> Sum4/1
  Sum4/1 -> Subsystem1/1(In1)
  Subsystem1/1(Out1) -> Sum2/2

== system main_SEPETC/active power sharing SE-PETC /EState_2/x2_o3 ==
  note: 利用x3对邻居的观测值，估计x3的状态
  Gain : Gain  Gain=cp
  Integrator : Integrator  ExternalReset=rising
  Subsystem1 : Subsystem
  Subsystem2 : Subsystem
  Subsystem3 : Subsystem
  Subsystem4 : Subsystem
  Sum2 : Sum  Inputs=|++
  Sum3 : Sum  Inputs=|++
  Sum4 : Sum  Inputs=|+-
  Sum5 : Sum  Inputs=|+-
  x2_o3 : Outport
  wires:
  Integrator/1 -> Sum3/1
  Sum3/1 -> Subsystem4/1(In1), Sum5/2, Sum4/2
  Gain/1 -> Integrator/1
  [x3_o4_hat] -> Sum4/1
  [x3_o2_hat] -> Sum5/1
  Sum5/1 -> Sum2/2
  Sum4/1 -> Sum2/1
  Sum2/1 -> Subsystem1/1(In1)
  Subsystem1/1(Out1) -> Gain/1
  [x3_hat] -> Subsystem2/1(In1)
  Subsystem2/1(Out1) -> Sum3/2
  [flag3] -> Subsystem3/1(In1)
  Subsystem3/1(Out1) -> Integrator/2
  Subsystem4/1(Out1) -> x2_o3/1

== system main_SEPETC/active power sharing SE-PETC /EState_3/x3_o2 ==
  Gain : Gain  Gain=cp
  Integrator : Integrator  ExternalReset=rising
  Subsystem1 : Subsystem
  Subsystem2 : Subsystem
  Subsystem3 : Subsystem
  Subsystem4 : Subsystem
  Sum : Sum  Inputs=|+-
  Sum2 : Sum  Inputs=|++
  Sum3 : Sum  Inputs=|++
  Sum4 : Sum  Inputs=|+-
  x3_o2 : Outport
  wires:
  Integrator/1 -> Sum3/1
  Sum3/1 -> Subsystem4/1(In1), Sum4/2, Sum/2
  Gain/1 -> Integrator/1
  [x2_o1_hat] -> Sum/1
  [x2_o3_hat] -> Sum4/1
  Sum4/1 -> Sum2/2
  Sum/1 -> Sum2/1
  Sum2/1 -> Subsystem1/1(In1)
  Subsystem1/1(Out1) -> Gain/1
  [flag2] -> Subsystem2/1(In1)
  Subsystem2/1(Out1) -> Integrator/2
  [x2_hat] -> Subsystem3/1(In1)
  Subsystem3/1(Out1) -> Sum3/2
  Subsystem4/1(Out1) -> x3_o2/1

== system main_SEPETC/active power sharing SE-PETC /EState_3/x3_o3 ==
  Gain : Gain  Gain=cp
  Integrator : Integrator  ExternalReset=rising
  Subsystem1 : Subsystem
  Subsystem2 : Subsystem
  Subsystem3 : Subsystem
  Subsystem4 : Subsystem
  Sum : Sum  Inputs=|+-
  Sum2 : Sum  Inputs=|++
  Sum3 : Sum  Inputs=|++
  Sum4 : Sum  Inputs=|+-
  x3_o3 : Outport
  wires:
  Sum/1 -> Sum2/1
  Integrator/1 -> Sum3/1
  Sum3/1 -> Subsystem4/1(In1), Sum4/2, Sum/2
  Gain/1 -> Integrator/1
  [x3_o2_hat] -> Sum/1
  [x3_o4_hat] -> Sum4/1
  Sum4/1 -> Sum2/2
  Sum2/1 -> Subsystem1/1(In1)
  Subsystem1/1(Out1) -> Gain/1
  [flag3] -> Subsystem2/1(In1)
  Subsystem2/1(Out1) -> Integrator/2
  [x3_hat] -> Subsystem3/1(In1)
  Subsystem3/1(Out1) -> Sum3/2
  Subsystem4/1(Out1) -> x3_o3/1

== system main_SEPETC/active power sharing SE-PETC /EState_3/x3_o4 ==
  note: 利用x4对邻居的观测值，估计x4的状态
  note: 利用x4对邻居的观测值，估计x4的状态
  Gain1 : Gain  Gain=cp
  Integrator1 : Integrator  ExternalReset=rising
  Subsystem1 : Subsystem
  Subsystem2 : Subsystem
  Subsystem3 : Subsystem
  Subsystem4 : Subsystem
  Sum : Sum  Inputs=|+-
  Sum5 : Sum  Inputs=|++
  Sum6 : Sum  Inputs=|++
  Sum7 : Sum  Inputs=|+-
  x3_o4 : Outport
  wires:
  Subsystem4/1(x3_o4) -> x3_o4/1
  Sum7/1 -> Sum5/2
  Gain1/1 -> Integrator1/1
  [x4_o1_hat] -> Sum/1
  [x4_o3_hat] -> Sum7/1
  Sum6/1 -> Subsystem4/1(In1), Sum7/2, Sum/2
  Sum/1 -> Sum5/1
  Integrator1/1 -> Sum6/1
  Sum5/1 -> Subsystem1/1(In1)
  Subsystem1/1(Out1) -> Gain1/1
  [flag4] -> Subsystem2/1(In1)
  Subsystem2/1(Out1) -> Integrator1/2
  [x4_hat] -> Subsystem3/1(In1)
  Subsystem3/1(Out1) -> Sum6/2

== system main_SEPETC/active power sharing SE-PETC /EState_4/x4_o1 ==
  note: 利用x1对邻居的观测值，估计x1的状态
  Gain1 : Gain  Gain=cp
  Integrator1 : Integrator  ExternalReset=rising
  Sum1 : Sum  Inputs=|+-
  Sum6 : Sum  Inputs=|++
  Sum7 : Sum  Inputs=|++
  Sum8 : Sum  Inputs=|+-
  x4_o1 : Outport
  wires:
  Sum8/1 -> Sum6/2
  [x1_o2_hat] -> Sum1/1
  [x1_o4_hat] -> Sum8/1
  Integrator1/1 -> Sum7/1
  Gain1/1 -> Integrator1/1
  Sum1/1 -> Sum6/1
  Sum6/1 -> Gain1/1
  [flag1] -> Integrator1/2
  [x1_hat] -> Sum7/2
  Sum7/1 -> x4_o1/1, Sum1/2, Sum8/2

== system main_SEPETC/active power sharing SE-PETC /EState_4/x4_o3 ==
  note: 利用x3对邻居的观测值，估计x3的状态
  Gain : Gain  Gain=cp
  Integrator : Integrator  ExternalReset=rising
  Subsystem1 : Subsystem
  Subsystem2 : Subsystem
  Subsystem3 : Subsystem
  Subsystem4 : Subsystem
  Sum : Sum  Inputs=|+-
  Sum2 : Sum  Inputs=|++
  Sum3 : Sum  Inputs=|++
  Sum4 : Sum  Inputs=|+-
  x4_o3 : Outport
  wires:
  Sum/1 -> Sum2/1
  Integrator/1 -> Sum3/1
  Sum3/1 -> Sum4/2, Sum/2, Subsystem3/1(In1)
  Gain/1 -> Integrator/1
  [x3_o4_hat] -> Sum4/1
  Sum4/1 -> Sum2/2
  [x3_o2_hat] -> Sum/1
  Sum2/1 -> Subsystem4/1(In1)
  Subsystem4/1(Out1) -> Gain/1
  [flag3] -> Subsystem1/1(In1)
  Subsystem1/1(Out1) -> Integrator/2
  [x3_hat] -> Subsystem2/1(In1)
  Subsystem2/1(Out1) -> Sum3/2
  Subsystem3/1(Out1) -> x4_o3/1

== system main_SEPETC/active power sharing SE-PETC /EState_4/x4_o4 ==
  Gain : Gain  Gain=cp
  Integrator : Integrator  ExternalReset=rising
  Subsystem1 : Subsystem
  Sum1 : Sum  Inputs=|++
  Sum2 : Sum  Inputs=|+-
  Sum3 : Sum  Inputs=|++
  Sum4 : Sum  Inputs=|+-
  x4_o4 : Outport
  wires:
  Integrator/1 -> Sum3/1
  [x4_hat] -> Sum3/2
  Sum3/1 -> Sum2/2, Sum4/2, x4_o4/1
  [flag4] -> Integrator/2
  Gain/1 -> Integrator/1
  [x4_o3_hat] -> Sum4/1
  Sum1/1 -> Gain/1
  [x4_o1_hat] -> Sum2/1
  Sum2/1 -> Sum1/1
  Sum4/1 -> Subsystem1/1(In1)
  Subsystem1/1(Out1) -> Sum1/2

== system main_SEPETC/active power sharing SE-PETC 1/EState_1/x1_o1 ==
  Gain : Gain  Gain=cp
  Integrator : Integrator  ExternalReset=rising
  Sum : Sum  Inputs=|+-
  Sum2 : Sum  Inputs=|++
  Sum3 : Sum  Inputs=|++
  Sum4 : Sum  Inputs=|+-
  x1_o1 : Outport
  wires:
  Integrator/1 -> Sum3/1
  [x1_hat] -> Sum3/2
  [flag1] -> Integrator/2
  Sum2/1 -> Gain/1
  Gain/1 -> Integrator/1
  [x1_o2_hat] -> Sum/1
  [x1_o4_hat] -> Sum4/1
  Sum3/1 -> Sum/2, Sum4/2, x1_o1/1
  Sum/1 -> Sum2/2
  Sum4/1 -> Sum2/1

== system main_SEPETC/active power sharing SE-PETC 1/EState_1/x1_o2 ==
  note: 利用x2对邻居的观测值，估计x2的状态
  Gain : Gain  Gain=cp
  Integrator : Integrator  ExternalReset=rising
  Subsystem1 : Subsystem
  Sum : Sum  Inputs=|+-
  Sum2 : Sum  Inputs=|++
  Sum3 : Sum  Inputs=|++
  Sum4 : Sum  Inputs=|+-
  x1_o2 : Outport
  wires:
  Sum/1 -> Sum2/1
  Integrator/1 -> Sum3/1
  Sum3/1 -> Sum4/2, Sum/2, x1_o2/1
  [flag2] -> Integrator/2
  Sum2/1 -> Gain/1
  Gain/1 -> Integrator/1
  [x2_o3_hat] -> Sum4/1
  [x2_o1_hat] -> Sum/1
  [x2_hat] -> Sum3/2
  Sum4/1 -> Subsystem1/1(In1)
  Subsystem1/1(Out1) -> Sum2/2

== system main_SEPETC/active power sharing SE-PETC 1/EState_1/x1_o4 ==
  note: 利用x4对邻居的观测值，估计x4的状态
  Gain : Gain  Gain=cp
  Integrator : Integrator  ExternalReset=rising
  Subsystem4 : Subsystem
  Sum : Sum  Inputs=|+-
  Sum2 : Sum  Inputs=|++
  Sum3 : Sum  Inputs=|++
  Sum4 : Sum  Inputs=|+-
  x1_o4 : Outport
  wires:
  Sum/1 -> Sum2/1
  Integrator/1 -> Sum3/1
  Sum3/1 -> x1_o4/1, Sum4/2, Sum/2
  Gain/1 -> Integrator/1
  [x4_o3_hat] -> Sum4/1
  [x4_o1_hat] -> Sum/1
  Sum2/1 -> Gain/1
  [x4_hat] -> Sum3/2
  [flag4] -> Integrator/2
  Sum4/1 -> Subsystem4/1(In1)
  Subsystem4/1(Out1) -> Sum2/2

== system main_SEPETC/active power sharing SE-PETC 1/EState_2/x2_o1 ==
  note: 利用x1对邻居的观测值，估计x1的状态
  Gain1 : Gain  Gain=cp
  Integrator1 : Integrator  ExternalReset=rising
  Sum4 : Sum  Inputs=|+-
  Sum6 : Sum  Inputs=|++
  Sum7 : Sum  Inputs=|++
  Sum8 : Sum  Inputs=|+-
  x2_o1 : Outport
  wires:
  Sum7/1 -> Sum8/2, Sum4/2, x2_o1/1
  Sum8/1 -> Sum6/2
  [x1_o2_hat] -> Sum4/1
  [x1_o4_hat] -> Sum8/1
  Integrator1/1 -> Sum7/1
  Sum6/1 -> Gain1/1
  [flag1] -> Integrator1/2
  Gain1/1 -> Integrator1/1
  [x1_hat] -> Sum7/2
  Sum4/1 -> Sum6/1

== system main_SEPETC/active power sharing SE-PETC 1/EState_2/x2_o2 ==
  Gain : Gain  Gain=cp
  Integrator : Integrator  ExternalReset=rising
  Subsystem1 : Subsystem
  Sum : Sum  Inputs=|+-
  Sum2 : Sum  Inputs=|++
  Sum3 : Sum  Inputs=|++
  Sum4 : Sum  Inputs=|+-
  x2_o2 : Outport
  wires:
  Sum/1 -> Sum2/1
  Integrator/1 -> Sum3/1
  [x2_hat] -> Sum3/2
  Sum3/1 -> Sum4/2, Sum/2, x2_o2/1
  [flag2] -> Integrator/2
  Sum2/1 -> Gain/1
  Gain/1 -> Integrator/1
  [x2_o1_hat] -> Sum/1
  [x2_o3_hat] -> Sum4/1
  Sum4/1 -> Subsystem1/1(In1)
  Subsystem1/1(Out1) -> Sum2/2

== system main_SEPETC/active power sharing SE-PETC 1/EState_2/x2_o3 ==
  note: 利用x3对邻居的观测值，估计x3的状态
  Gain : Gain  Gain=cp
  Integrator : Integrator  ExternalReset=rising
  Subsystem1 : Subsystem
  Subsystem2 : Subsystem
  Subsystem3 : Subsystem
  Subsystem4 : Subsystem
  Sum2 : Sum  Inputs=|++
  Sum3 : Sum  Inputs=|++
  Sum4 : Sum  Inputs=|+-
  Sum5 : Sum  Inputs=|+-
  x2_o3 : Outport
  wires:
  Integrator/1 -> Sum3/1
  Sum3/1 -> Subsystem4/1(In1), Sum5/2, Sum4/2
  Gain/1 -> Integrator/1
  [x3_o4_hat] -> Sum4/1
  [x3_o2_hat] -> Sum5/1
  Sum5/1 -> Sum2/2
  Sum4/1 -> Sum2/1
  Sum2/1 -> Subsystem1/1(In1)
  Subsystem1/1(Out1) -> Gain/1
  [x3_hat] -> Subsystem2/1(In1)
  Subsystem2/1(Out1) -> Sum3/2
  [flag3] -> Subsystem3/1(In1)
  Subsystem3/1(Out1) -> Integrator/2
  Subsystem4/1(Out1) -> x2_o3/1

== system main_SEPETC/active power sharing SE-PETC 1/EState_3/x3_o2 ==
  Gain : Gain  Gain=cp
  Integrator : Integrator  ExternalReset=rising
  Subsystem1 : Subsystem
  Subsystem2 : Subsystem
  Subsystem3 : Subsystem
  Subsystem4 : Subsystem
  Sum : Sum  Inputs=|+-
  Sum2 : Sum  Inputs=|++
  Sum3 : Sum  Inputs=|++
  Sum4 : Sum  Inputs=|+-
  x3_o2 : Outport
  wires:
  Integrator/1 -> Sum3/1
  Sum3/1 -> Subsystem4/1(In1), Sum4/2, Sum/2
  Gain/1 -> Integrator/1
  [x2_o1_hat] -> Sum/1
  [x2_o3_hat] -> Sum4/1
  Sum4/1 -> Sum2/2
  Sum/1 -> Sum2/1
  Sum2/1 -> Subsystem1/1(In1)
  Subsystem1/1(Out1) -> Gain/1
  [flag2] -> Subsystem2/1(In1)
  Subsystem2/1(Out1) -> Integrator/2
  [x2_hat] -> Subsystem3/1(In1)
  Subsystem3/1(Out1) -> Sum3/2
  Subsystem4/1(Out1) -> x3_o2/1

== system main_SEPETC/active power sharing SE-PETC 1/EState_3/x3_o3 ==
  Gain : Gain  Gain=cp
  Integrator : Integrator  ExternalReset=rising
  Subsystem1 : Subsystem
  Subsystem2 : Subsystem
  Subsystem3 : Subsystem
  Subsystem4 : Subsystem
  Sum : Sum  Inputs=|+-
  Sum2 : Sum  Inputs=|++
  Sum3 : Sum  Inputs=|++
  Sum4 : Sum  Inputs=|+-
  x3_o3 : Outport
  wires:
  Sum/1 -> Sum2/1
  Integrator/1 -> Sum3/1
  Sum3/1 -> Subsystem4/1(In1), Sum4/2, Sum/2
  Gain/1 -> Integrator/1
  [x3_o2_hat] -> Sum/1
  [x3_o4_hat] -> Sum4/1
  Sum4/1 -> Sum2/2
  Sum2/1 -> Subsystem1/1(In1)
  Subsystem1/1(Out1) -> Gain/1
  [flag3] -> Subsystem2/1(In1)
  Subsystem2/1(Out1) -> Integrator/2
  [x3_hat] -> Subsystem3/1(In1)
  Subsystem3/1(Out1) -> Sum3/2
  Subsystem4/1(Out1) -> x3_o3/1

== system main_SEPETC/active power sharing SE-PETC 1/EState_3/x3_o4 ==
  note: 利用x4对邻居的观测值，估计x4的状态
  note: 利用x4对邻居的观测值，估计x4的状态
  Gain1 : Gain  Gain=cp
  Integrator1 : Integrator  ExternalReset=rising
  Subsystem1 : Subsystem
  Subsystem2 : Subsystem
  Subsystem3 : Subsystem
  Subsystem4 : Subsystem
  Sum : Sum  Inputs=|+-
  Sum5 : Sum  Inputs=|++
  Sum6 : Sum  Inputs=|++
  Sum7 : Sum  Inputs=|+-
  x3_o4 : Outport
  wires:
  Subsystem4/1(x3_o4) -> x3_o4/1
  Sum7/1 -> Sum5/2
  Gain1/1 -> Integrator1/1
  [x4_o1_hat] -> Sum/1
  [x4_o3_hat] -> Sum7/1
  Sum6/1 -> Subsystem4/1(In1), Sum7/2, Sum/2
  Sum/1 -> Sum5/1
  Integrator1/1 -> Sum6/1
  Sum5/1 -> Subsystem1/1(In1)
  Subsystem1/1(Out1) -> Gain1/1
  [flag4] -> Subsystem2/1(In1)
  Subsystem2/1(Out1) -> Integrator1/2
  [x4_hat] -> Subsystem3/1(In1)
  Subsystem3/1(Out1) -> Sum6/2

== system main_SEPETC/active power sharing SE-PETC 1/EState_4/x4_o1 ==
  note: 利用x1对邻居的观测值，估计x1的状态
  Gain1 : Gain  Gain=cp
  Integrator1 : Integrator  ExternalReset=rising
  Sum1 : Sum  Inputs=|+-
  Sum6 : Sum  Inputs=|++
  Sum7 : Sum  Inputs=|++
  Sum8 : Sum  Inputs=|+-
  x4_o1 : Outport
  wires:
  Sum8/1 -> Sum6/2
  [x1_o2_hat] -> Sum1/1
  [x1_o4_hat] -> Sum8/1
  Integrator1/1 -> Sum7/1
  Gain1/1 -> Integrator1/1
  Sum1/1 -> Sum6/1
  Sum6/1 -> Gain1/1
  [flag1] -> Integrator1/2
  [x1_hat] -> Sum7/2
  Sum7/1 -> x4_o1/1, Sum1/2, Sum8/2

== system main_SEPETC/active power sharing SE-PETC 1/EState_4/x4_o3 ==
  note: 利用x3对邻居的观测值，估计x3的状态
  Gain : Gain  Gain=cp
  Integrator : Integrator  ExternalReset=rising
  Subsystem1 : Subsystem
  Subsystem2 : Subsystem
  Subsystem3 : Subsystem
  Subsystem4 : Subsystem
  Sum : Sum  Inputs=|+-
  Sum2 : Sum  Inputs=|++
  Sum3 : Sum  Inputs=|++
  Sum4 : Sum  Inputs=|+-
  x4_o3 : Outport
  wires:
  Sum/1 -> Sum2/1
  Integrator/1 -> Sum3/1
  Sum3/1 -> Sum4/2, Sum/2, Subsystem3/1(In1)
  Gain/1 -> Integrator/1
  [x3_o4_hat] -> Sum4/1
  Sum4/1 -> Sum2/2
  [x3_o2_hat] -> Sum/1
  Sum2/1 -> Subsystem4/1(In1)
  Subsystem4/1(Out1) -> Gain/1
  [flag3] -> Subsystem1/1(In1)
  Subsystem1/1(Out1) -> Integrator/2
  [x3_hat] -> Subsystem2/1(In1)
  Subsystem2/1(Out1) -> Sum3/2
  Subsystem3/1(Out1) -> x4_o3/1

== system main_SEPETC/active power sharing SE-PETC 1/EState_4/x4_o4 ==
  Gain : Gain  Gain=cp
  Integrator : Integrator  ExternalReset=rising
  Subsystem1 : Subsystem
  Sum1 : Sum  Inputs=|++
  Sum2 : Sum  Inputs=|+-
  Sum3 : Sum  Inputs=|++
  Sum4 : Sum  Inputs=|+-
  x4_o4 : Outport
  wires:
  Integrator/1 -> Sum3/1
  [x4_hat] -> Sum3/2
  Sum3/1 -> Sum2/2, Sum4/2, x4_o4/1
  [flag4] -> Integrator/2
  Gain/1 -> Integrator/1
  [x4_o3_hat] -> Sum4/1
  Sum1/1 -> Gain/1
  [x4_o1_hat] -> Sum2/1
  Sum2/1 -> Sum1/1
  Sum4/1 -> Subsystem1/1(In1)
  Subsystem1/1(Out1) -> Sum1/2

== system main_SEPETC/controller 1/(P) abc to dq2/abc to Alpha-Beta-Zero ==
  abc : Inport  PortDimensions=3
  Gain1 : Gain  Gain=sqrt(2/3)  SaturateOnIntegerOverflow=on  OutDataTypeStr=Inherit: Same as input  ParamDataTypeStr=Inherit: Same as input
  Gain3 : Gain  Gain="[ 1   -1/2   -1/2; 0   sqrt(3)/2   -sqrt(3)/2; 1/sqrt(2)  1/sqrt(2)  1/sqrt(2) ]"  Multiplication=Matrix(K*u) (u vector)  SaturateOnIntegerOverflow=on  OutDataTypeStr=Inherit: Same as input  ParamDataTypeStr=Inherit: Same as input
  al_be_0 : Outport  VectorParamsAs1DForOutWhenUnconnected=off
  wires:
  abc/1 -> Gain3/1
  Gain3/1 -> Gain1/1
  Gain1/1 -> al_be_0/1

== system main_SEPETC/controller 1/primary 1/(P) abc to dq1 ==
  abc : Inport  PortDimensions=3
  wt : Inport  Port=2  PortDimensions=1
  Alpha-Beta-Zero to dq0 : spsAlphaBetaZerotodq0Lib/Alpha-Beta-Zero to dq0  Alignment=90 degrees behind phase A axis
      settings: SourceProductBaseCode=PS
  abc to Alpha-Beta-Zero : Subsystem  AncestorBlock=powerlib_meascontrol/Transformations/abc to Alpha-Beta-Zero  DialogController=POWERSYS.PowerSysDialog  LoadFcn=sps_rtmsupport('LoadFcn', gcbh);  StartFcn=sps_rtmsupport('StartFcn', gcbh);  StopFcn=sps_rtmsupport('StopFcn', gcbh);  mask(abc to Alpha-Beta-Zero Transformation){}
      mask help: Perform a Clarke transformation from a three-phase (abc) signal to a alpha-beta-zero stationary reference frame.
      settings: CopyFcn=sps_rtmsupport('CopyFcn', gcbh);  DeleteFcn=sps_rtmsupport('DeleteFcn', gcbh);  UndoDeleteFcn=sps_rtmsupport('UndoDeleteFcn', gcbh);  ModelCloseFcn=sps_rtmsupport('ModelCloseFcn', gcbh);  PreSaveFcn=sps_rtmsupport('PreSaveFcn', gcbh);  PostSaveFcn=sps_rtmsupport('PostSaveFcn', gcbh);  NameChangeFcn=sps_rtmsupport('NameChangeFcn', gcbh);  PreCopyFcn=sps_rtmsupport('PreCopyFcn', gcbh);  OpenFcn=sps_rtmsupport('OpenFcn', gcbh, []);  CloseFcn=sps_rtmsupport('CloseFcn', gcbh);  PreDeleteFcn=sps_rtmsupport('PreDeleteFcn', gcbh);
      mask Help: helpview(psbhelp);
      mask Display:
      | plot([0 1], [0,1])
      | text(0.15,0.7,'abc')
      | text(0.55, 0.3,'\alpha\beta0','texmode','on')
  dq0 : Outport  VectorParamsAs1DForOutWhenUnconnected=off
  wires:
  wt/1 -> Alpha-Beta-Zero to dq0/2
  abc/1 -> abc to Alpha-Beta-Zero/1(abc)
  Alpha-Beta-Zero to dq0/1 -> dq0/1
  abc to Alpha-Beta-Zero/1(al_be_0) -> Alpha-Beta-Zero to dq0/1
